simulink model "ejercicio1"  (R2018a)
settings: Solver=VariableStepAuto  StartTime=0.0  StopTime=20.0  RelTol=1e-3
settings Model: Creator=OSCAR  LastModifiedBy=OSCAR

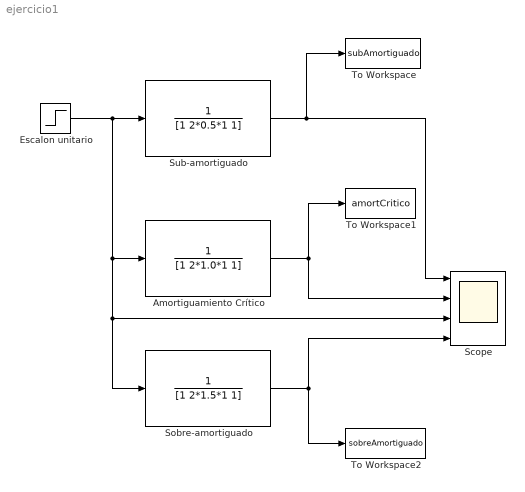
== system ejercicio1 ==
  " Sobre-amortiguado" : TransferFcn  Denominator=[1 2*1.5*1 1]
  Amortiguamiento Crítico : TransferFcn  Denominator=[1 2*1.0*1 1]
  Escalon unitario : Step  SampleTime=0.01
  Scope : Scope  NumInputPorts=4
  Sub-amortiguado : TransferFcn  Denominator=[1 2*0.5*1 1]
  To Workspace : ToWorkspace  VariableName=subAmortiguado  SampleTime=-1
  To Workspace1 : ToWorkspace  VariableName=amortCritico  SampleTime=-1
  To Workspace2 : ToWorkspace  VariableName=sobreAmortiguado  SampleTime=-1
  wires:
  Escalon unitario/1 -> Scope/3, " Sobre-amortiguado"/1, Amortiguamiento Crítico/1, Sub-amortiguado/1
  Sub-amortiguado/1 -> Scope/1, To Workspace/1
  " Sobre-amortiguado"/1 -> Scope/4, To Workspace2/1
  Amortiguamiento Crítico/1 -> Scope/2, To Workspace1/1
